simulink library "CtrlSurfMapping_Lib"  (Simulink 8.4)
settings: Solver=ode45  StartTime=0.0  StopTime=10.0  RelTol=1e-3
undefined symbols (not defined in the file): AC
libraries: CtrlSurfMapping_Lib x1
settings Model: Creator=hpfifer  LastModifiedBy=pseiler

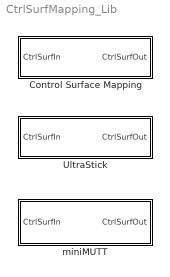
== system CtrlSurfMapping_Lib ==
  Control Surface Mapping : Subsystem  BlockChoice=UltraStick  mask{aircraft=AC.aircraft}
      mask prompts: aircraft "Aircraft type:"
      mask init:
      | pathname = gcb;
      | 
      | switch lower(aircraft)
      |     case 'ultrastick120'
      |         set_param(pathname,'BlockChoice','UltraStick');
      |    case 'ultrastick25e'
      |         set_param(pathname,'BlockChoice','UltraStick');
      |     case 'minimutt'
      |         set_param(pathname,'BlockChoice','miniMUTT');
      | end
      settings: TemplateBlock=self  MemberBlocks=UltraStick,miniMUTT
  UltraStick : Subsystem
  miniMUTT : Subsystem

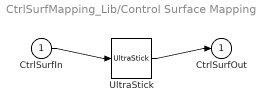
== system CtrlSurfMapping_Lib/Control Surface Mapping ==
  CtrlSurfIn : Inport
  UltraStick : CtrlSurfMapping_Lib/UltraStick
  CtrlSurfOut : Outport
  wires:
  CtrlSurfIn/1 -> UltraStick/1
  UltraStick/1 -> CtrlSurfOut/1

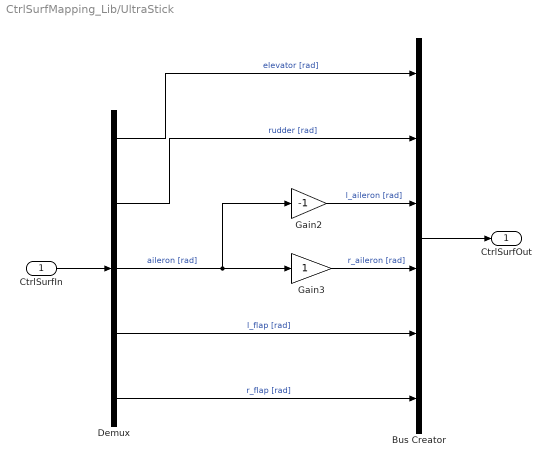
== system CtrlSurfMapping_Lib/UltraStick ==
  CtrlSurfIn : Inport
  Bus Creator : BusCreator  Inputs=6
  Demux : Demux  Outputs=5
  Gain2 : Gain  Gain=-1
  Gain3 : Gain
  CtrlSurfOut : Outport
  wires:
  CtrlSurfIn/1 -> Demux/1
  Bus Creator/1 -> CtrlSurfOut/1
  Demux/3 -> Gain2/1, Gain3/1  "aileron [rad]"
  Gain2/1 -> Bus Creator/3  "l_aileron [rad]"
  Gain3/1 -> Bus Creator/4  "r_aileron [rad]"
  Demux/1 -> Bus Creator/1  "elevator [rad]"
  Demux/4 -> Bus Creator/5  "l_flap [rad]"
  Demux/5 -> Bus Creator/6  "r_flap [rad]"
  Demux/2 -> Bus Creator/2  "rudder [rad]"

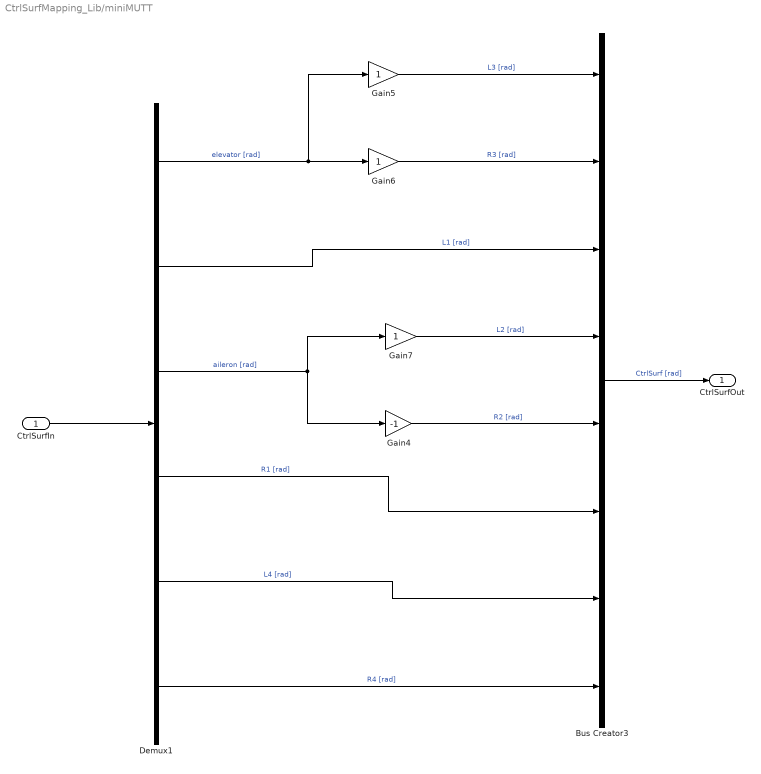
== system CtrlSurfMapping_Lib/miniMUTT ==
  CtrlSurfIn : Inport
  Bus Creator3 : BusCreator  Inputs=8
  Demux1 : Demux  Outputs=6
  Gain4 : Gain  Gain=-1
  Gain5 : Gain
  Gain6 : Gain
  Gain7 : Gain
  CtrlSurfOut : Outport
  wires:
  Bus Creator3/1 -> CtrlSurfOut/1  "CtrlSurf [rad]"
  Gain5/1 -> Bus Creator3/1  "L3 [rad]"
  Gain6/1 -> Bus Creator3/2  "R3 [rad]"
  Demux1/1 -> Gain5/1, Gain6/1  "elevator [rad]"
  Demux1/2 -> Bus Creator3/3  "L1 [rad]"
  Gain7/1 -> Bus Creator3/4  "L2 [rad]"
  Gain4/1 -> Bus Creator3/5  "R2 [rad]"
  Demux1/3 -> Gain7/1, Gain4/1  "aileron [rad]"
  Demux1/6 -> Bus Creator3/8  "R4 [rad]"
  Demux1/5 -> Bus Creator3/7  "L4 [rad]"
  Demux1/4 -> Bus Creator3/6  "R1 [rad]"
  CtrlSurfIn/1 -> Demux1/1
